simulink model "Brk"  (R2020b)
settings: configuration reference "gen_config" (kept outside this file)
settings Model: DataDictionary=Hybrid_vehicle.sldd  SimulationMode=accelerator  Creator=Georg  LastModifiedBy=jy
settings ConfigSetRef: SourceName=gen_config

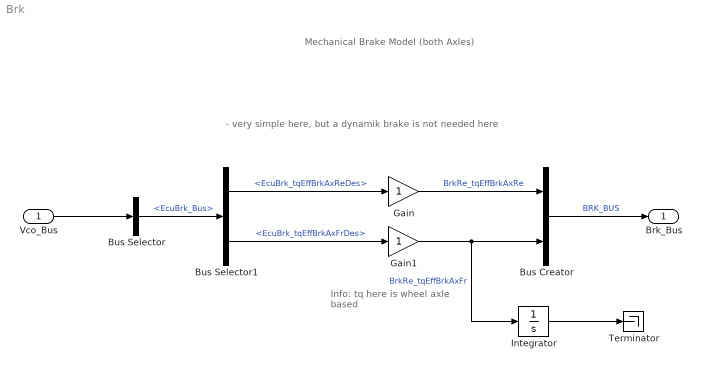
== system Brk ==
  note: Info:
      | tq here is wheel axle based
  note: - very simple here, but a dynamik brake is not needed here
  note: Mechanical Brake Model
      | (both Axles)
  Vco_Bus : Inport  OutDataTypeStr=Bus: VCO_BUS  BusOutputAsStruct=on
  Bus Creator : BusCreator  Inputs=2  OutDataTypeStr=Bus: BRK_BUS  NonVirtualBus=on
  Bus Selector : BusSelector  OutputSignals=EcuBrk_Bus
  Bus Selector1 : BusSelector  OutputSignals=EcuBrk_tqEffBrkAxReDes,EcuBrk_tqEffBrkAxFrDes
  Gain : Gain
  Gain1 : Gain
  Integrator : Integrator
  Terminator : Terminator
  Brk_Bus : Outport  OutDataTypeStr=Bus: BRK_BUS  VectorParamsAs1DForOutWhenUnconnected=off
  wires:
  Bus Creator/1 -> Brk_Bus/1  "BRK_BUS"
  Bus Selector1/1 -> Gain/1  "<EcuBrk_tqEffBrkAxReDes>"
  Gain/1 -> Bus Creator/1  "BrkRe_tqEffBrkAxRe"
  Bus Selector1/2 -> Gain1/1  "<EcuBrk_tqEffBrkAxFrDes>"
  Bus Selector/1 -> Bus Selector1/1  "<EcuBrk_Bus>"
  Vco_Bus/1 -> Bus Selector/1
  Gain1/1 -> Integrator/1, Bus Creator/2  "BrkRe_tqEffBrkAxFr"
  Integrator/1 -> Terminator/1
